simulink subsystem "SimulinkModel"  (R2023a)
settings: Solver=VariableStepAuto  StartTime=0.0  StopTime=10.0  RelTol=1e-3
undefined symbols (not defined in the file): c
settings Model: Creator=is123  LastModifiedBy=is123
settings OptimizationCC: ReuseModelBlockBuffer=off

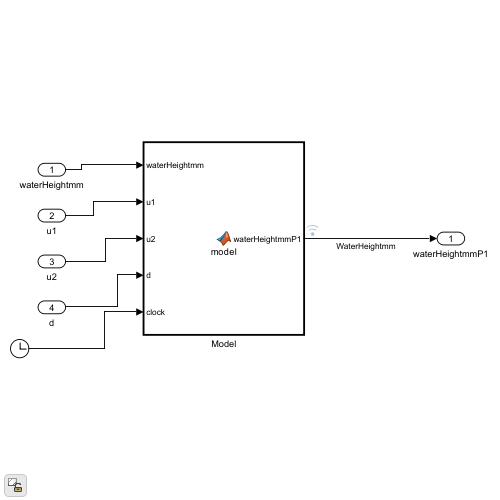
[thumbnail: Simulink's stored preview of the top-level diagram]
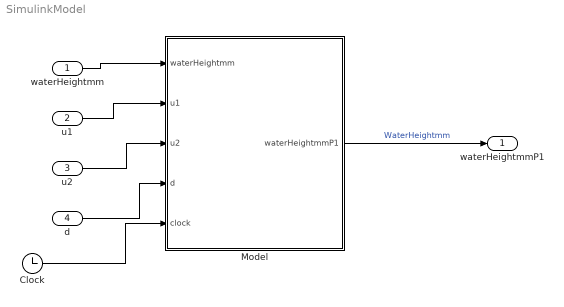
== system SimulinkModel ==
  waterHeightmm : Inport
  u1 : Inport  Port=2
  u2 : Inport  Port=3
  d : Inport  Port=4
  Clock : Clock
  Model : MATLAB Function  TreatAsAtomicUnit=on  SystemSampleTime=3600/c.AccTime
  waterHeightmmP1 : Outport
  wires:
  waterHeightmm/1 -> Model/1(waterHeightmm)
  u1/1 -> Model/2(u1)
  d/1 -> Model/4(d)
  u2/1 -> Model/3(u2)
  Model/1(waterHeightmmP1) -> waterHeightmmP1/1  "WaterHeightmm"
  Clock/1 -> Model/5(clock)

== matlab function SimulinkModel/Model ==
  data: waterHeightmm input; u1 input; u2 input; waterHeightmmP1 output; d input; clock input
function waterHeightmmP1 = model(waterHeightmm,u1,u2,d,clock)
%Determining the next water height in the water tower. 

if clock <200 
    waterHeightmmP1=waterHeightmm; 
else 
%Setting the output to zero becuase it is needed
waterHeightmmP1=zeros(1,1);

%loading in scaled standard constants 
c=scaled_standard_constants;

%Collecting the used mass flows into a vector 
u=[u1;u2];

%Determine the water volume instead of water height 
V=waterHeightmm/1e3*c.At;

%calling the model function to get the next volumen
Vp1=Model(V,u,d);

%Determine water height instead of water volume: 
waterHeightmmP1=Vp1/c.At*1e3; 
end 
end
